simulink model "aero_ground_model"  (R2013b)
settings: Solver=ode23  StartTime=0.0  StopTime=100  FixedStep=0.01  MaxStep=1  RelTol=1e-3
undefined symbols (not defined in the file or in its folder): par
libraries: simulink x12, coeffs x3, lateral_model x3, dspswit3 x1
(part 2 of 2)

== system aero_ground_model/Physical Model/Tire Forces/Wheels Velocity/Velocity_L ==
  STATE : Inport
  " " : Constant  Value=par.l_yL
  "  " : Constant  Value=par.l_xL
  Add : Sum
  Add1 : Sum  Inputs=+-
  Bus Creator : BusCreator  Inputs=2
  Bus Selector : BusSelector  OutputSignals=[Vx; Vy],Wz
  Bus Selector1 : BusSelector  OutputSignals=v_X,v_Y
  Product : Product
  Product1 : Product
  V_L : Outport
  wires:
  STATE/1 -> Bus Selector/1
  Bus Selector/1 -> Bus Selector1/1  "<[Vx; Vy]>"
  Bus Selector1/1 -> Add/1  "<v_X>"
  Bus Selector/2 -> Product1/1, Product/2  "<Wz>"
  " "/1 -> Product/1
  Product/1 -> Add/2
  Product1/1 -> Add1/2
  Bus Selector1/2 -> Add1/1  "<v_Y>"
  "  "/1 -> Product1/2
  Add1/1 -> Bus Creator/2  "V_y"
  Add/1 -> Bus Creator/1  "V_x"
  Bus Creator/1 -> V_L/1

== system aero_ground_model/Physical Model/Tire Forces/Wheels Velocity/Velocity_N ==
  note: V_N = f(V,W)
  note: 1. Vx_N = Vx * cos(delta) + (Vy + l_xN * Wz) * sin(delta)
      |
      | 2. Vy_N = (Vx + l_xN * Wz) * cos(delta) - Vx * sin(delta)
  STATE : Inport
  delta : Inport  Port=2
  Bus Creator : BusCreator  Inputs=2
  Bus Selector : BusSelector  OutputSignals=[Vx; Vy],Wz
  Bus Selector1 : BusSelector  OutputSignals=v_X,v_Y
  VxN : Subsystem
  VyN : Subsystem
  V_N : Outport
  wires:
  STATE/1 -> Bus Selector/1
  Bus Selector/1 -> Bus Selector1/1  "<[Vx; Vy]>"
  VyN/1(VyN) -> Bus Creator/2  "V_y"
  Bus Creator/1 -> V_N/1
  delta/1 -> VyN/1(delta), VxN/1(delta)
  Bus Selector1/1 -> VyN/2(Vx), VxN/2(Vx)  "<v_X>"
  Bus Selector1/2 -> VyN/3(Vy), VxN/3(Vy)  "<v_Y>"
  Bus Selector/2 -> VyN/4(Wz), VxN/4(Wz)  "<Wz>"
  VxN/1(VxN) -> Bus Creator/1  "V_x"

== system aero_ground_model/Physical Model/Tire Forces/Wheels Velocity/Velocity_R ==
  STATE : Inport
  " " : Constant  Value=par.l_yR
  "  " : Constant  Value=par.l_xR
  Add : Sum  Inputs=+-
  Add1 : Sum  Inputs=+-
  Bus Creator : BusCreator  Inputs=2
  Bus Selector : BusSelector  OutputSignals=[Vx; Vy],Wz
  Bus Selector1 : BusSelector  OutputSignals=v_X,v_Y
  Product : Product
  Product1 : Product
  V_R : Outport
  wires:
  STATE/1 -> Bus Selector/1
  Bus Selector/1 -> Bus Selector1/1  "<[Vx; Vy]>"
  Bus Selector1/1 -> Add/1  "<v_X>"
  Bus Selector/2 -> Product1/1, Product/2  "<Wz>"
  " "/1 -> Product/1
  Product/1 -> Add/2
  Product1/1 -> Add1/2
  Bus Selector1/2 -> Add1/1  "<v_Y>"
  "  "/1 -> Product1/2
  Add1/1 -> Bus Creator/2  "V_y"
  Add/1 -> Bus Creator/1  "V_x"
  Bus Creator/1 -> V_R/1

== system aero_ground_model/Physical Model/Forces to Velocities/Velocity/velo_X/F_xN * cos(delta) ==
  F_xN : Inport
  delta : Inport  Port=2
  Projection of nose-wheel resistance force into X axis : Product
  Trigonometric Function : Trigonometry  Operator=cos
  Out1 : Outport
  wires:
  F_xN/1 -> Projection of nose-wheel resistance force into X axis/1
  Trigonometric Function/1 -> Projection of nose-wheel resistance force into X axis/2
  Projection of nose-wheel resistance force into X axis/1 -> Out1/1
  delta/1 -> Trigonometric Function/1

== system aero_ground_model/Physical Model/Forces to Velocities/Velocity/velo_X/F_yN * sin(delta) ==
  delta : Inport
  F_yN : Inport  Port=2
  Projection of nose-wheel lateral force into X-axis : Product
  Trigonometric Function : Trigonometry
  Out1 : Outport
  wires:
  F_yN/1 -> Projection of nose-wheel lateral force into X-axis/1
  Trigonometric Function/1 -> Projection of nose-wheel lateral force into X-axis/2
  Projection of nose-wheel lateral force into X-axis/1 -> Out1/1
  delta/1 -> Trigonometric Function/1

== system aero_ground_model/Physical Model/Forces to Velocities/Velocity/velo_Y/*cos(delta) ==
  delta : Inport
  F_yN : Inport  Port=2
  Projection of nose-wheel lateral force into Y axis : Product
  Trigonometric Function : Trigonometry  Operator=cos
  Out1 : Outport
  wires:
  F_yN/1 -> Projection of nose-wheel lateral force into Y axis/1
  Trigonometric Function/1 -> Projection of nose-wheel lateral force into Y axis/2
  Projection of nose-wheel lateral force into Y axis/1 -> Out1/1
  delta/1 -> Trigonometric Function/1

== system aero_ground_model/Physical Model/Forces to Velocities/Velocity/velo_Y/*sin(delta) ==
  delta : Inport
  F_xN : Inport  Port=2
  Projection of nose-wheel resistance force into Y-axis : Product
  Trigonometric Function : Trigonometry
  Out1 : Outport
  wires:
  Trigonometric Function/1 -> Projection of nose-wheel resistance force into Y-axis/2
  Projection of nose-wheel resistance force into Y-axis/1 -> Out1/1
  delta/1 -> Trigonometric Function/1
  F_xN/1 -> Projection of nose-wheel resistance force into Y-axis/1

== system aero_ground_model/Physical Model/Tire Forces/Lateral tire Force/Slip Angles/arctan(V_L) ==
  note: Slip Angle
  note: alpha = arctan(Vy/Vx)
  V : Inport
  Bus Selector : BusSelector  OutputSignals=V_y,V_x
  Trigonometric Function : Trigonometry  Operator=atan2
  atan(V) : Outport
  wires:
  V/1 -> Bus Selector/1
  Bus Selector/2 -> Trigonometric Function/2  "<V_x>"
  Bus Selector/1 -> Trigonometric Function/1  "<V_y>"
  Trigonometric Function/1 -> atan(V)/1

== system aero_ground_model/Physical Model/Tire Forces/Lateral tire Force/Slip Angles/arctan(V_N) ==
  note: Slip Angle
  note: alpha = arctan(Vy/Vx)
  V : Inport
  Bus Selector : BusSelector  OutputSignals=V_y,V_x
  Trigonometric Function : Trigonometry  Operator=atan2
  atan(V) : Outport
  wires:
  V/1 -> Bus Selector/1
  Bus Selector/2 -> Trigonometric Function/2  "<V_x>"
  Trigonometric Function/1 -> atan(V)/1
  Bus Selector/1 -> Trigonometric Function/1  "<V_y>"

== system aero_ground_model/Physical Model/Tire Forces/Lateral tire Force/Slip Angles/arctan(V_R) ==
  note: Slip Angle
  note: alpha = arctan(Vy/Vx)
  V : Inport
  Bus Selector : BusSelector  OutputSignals=V_y,V_x
  Trigonometric Function : Trigonometry  Operator=atan2
  atan(V) : Outport
  wires:
  V/1 -> Bus Selector/1
  Bus Selector/2 -> Trigonometric Function/2  "<V_x>"
  Trigonometric Function/1 -> atan(V)/1
  Bus Selector/1 -> Trigonometric Function/1  "<V_y>"

== system aero_ground_model/Physical Model/Tire Forces/Longitudal Tire Force/Braking/L brake ==
  note: brakes - ratio of brakes being applied (0-1)
      | mu_Beff - friction coeff., effectivity of ABS braking system
  note: Model of simple ABS brakes
  F_zRL : Inport
  environ : Inport  Port=2
  brakes : Inport  Port=3
  Bus Selector : BusSelector  OutputSignals=coeffs_L.mu_Beff
  Gain : Gain  Gain=0.3
  Product : Product
  Product1 : Product
  F_xL : Outport
  wires:
  environ/1 -> Bus Selector/1
  Bus Selector/1 -> Product/2  "<mu_Beff>"
  F_zRL/1 -> Product/1
  brakes/1 -> Product1/1
  Product/1 -> Product1/2
  Product1/1 -> Gain/1
  Gain/1 -> F_xL/1

== system aero_ground_model/Physical Model/Tire Forces/Longitudal Tire Force/Braking/R brake ==
  note: brakes - ratio of brakes being applied (0-1)
      | mu_Beff - friction coeff., effectivity of ABS braking system
  note: Model of simple ABS brakes
  brakes : Inport
  F_zRL : Inport  Port=2
  environ : Inport  Port=3
  Bus Selector : BusSelector  OutputSignals=coeffs_R.mu_Beff
  Gain : Gain  Gain=0.3
  Product : Product
  Product1 : Product
  F_xR : Outport
  wires:
  environ/1 -> Bus Selector/1
  Bus Selector/1 -> Product/2  "<mu_Beff>"
  F_zRL/1 -> Product/1
  Product/1 -> Product1/2
  brakes/1 -> Product1/1
  Product1/1 -> Gain/1
  Gain/1 -> F_xR/1

== system aero_ground_model/Physical Model/Tire Forces/Longitudal Tire Force/Rolling Resistance/Resist_L ==
  note: F_xL = mu_R * F_zL * (vL / v_thresh)
  note: Rolling Resistance of Left Tire
  coeffs : Inport
  F_zL : Inport  Port=2
  Bus Selector : BusSelector  OutputSignals=mu_R
  Product : Product
  F_xL : Outport
  wires:
  F_zL/1 -> Product/1
  Bus Selector/1 -> Product/2  "<mu_R>"
  coeffs/1 -> Bus Selector/1
  Product/1 -> F_xL/1

== system aero_ground_model/Physical Model/Tire Forces/Longitudal Tire Force/Rolling Resistance/Resist_N ==
  note: F_xN = mu_R * F_zN * (v / v_thresh)
  note: Rolling Resistance of Nose-Wheel Tire
  F_zN : Inport
  coeffs : Inport  Port=2
  Bus Selector : BusSelector  OutputSignals=mu_R
  Product : Product
  F_xN : Outport
  wires:
  F_zN/1 -> Product/1
  Bus Selector/1 -> Product/2  "<mu_R>"
  coeffs/1 -> Bus Selector/1
  Product/1 -> F_xN/1

== system aero_ground_model/Physical Model/Tire Forces/Longitudal Tire Force/Rolling Resistance/Resist_R ==
  note: (vR / v_thresh) limited to range 0-1
      | used to eliminate resistance forces
      | when plane stands still
  note: F_xR = mu_R * F_zR * (vR / v_thresh)
  note: Rolling Resistance of Right Tire
  F_zR : Inport
  coeffs : Inport  Port=2
  Bus Selector : BusSelector  OutputSignals=mu_R
  Product : Product
  F_xR : Outport
  wires:
  F_zR/1 -> Product/1
  Bus Selector/1 -> Product/2  "<mu_R>"
  coeffs/1 -> Bus Selector/1
  Product/1 -> F_xR/1

== system aero_ground_model/Physical Model/Tire Forces/Wheels Velocity/Velocity_N/VxN ==
  delta : Inport
  Vx : Inport  Port=2
  Vy : Inport  Port=3
  Wz : Inport  Port=4
  "     " : Constant  Value=par.l_xN
  Add : Sum
  Add2 : Sum
  Gain1 : Gain  Commented=on  Gain=-1
  Product1 : Product
  Product2 : Product
  Product3 : Product
  Trigonometric Function : Trigonometry  Operator=cos
  Trigonometric Function1 : Trigonometry
  VxN : Outport
  wires:
  Product3/1 -> Add/2
  Add/1 -> VxN/1  "V_x"
  Add2/1 -> Product3/2
  delta/1 -> Trigonometric Function/1, Trigonometric Function1/1
  Wz/1 -> Product1/2
  Product2/1 -> Add/1
  Trigonometric Function1/1 -> Product3/1
  Product1/1 -> Add2/2
  "     "/1 -> Product1/1
  Trigonometric Function/1 -> Product2/2
  Vx/1 -> Product2/1
  Vy/1 -> Add2/1

== system aero_ground_model/Physical Model/Tire Forces/Wheels Velocity/Velocity_N/VyN ==
  delta : Inport
  Vx : Inport  Port=2
  Vy : Inport  Port=3
  Wz : Inport  Port=4
  "     " : Constant  Value=par.l_xN
  Add : Sum  Inputs=-+
  Add2 : Sum
  Product1 : Product
  Product2 : Product
  Product3 : Product
  Trigonometric Function : Trigonometry
  Trigonometric Function1 : Trigonometry  Operator=cos
  VyN : Outport
  wires:
  Vy/1 -> Add2/1
  Product3/1 -> Add/2
  Add/1 -> VyN/1  "V_y"
  Add2/1 -> Product3/2
  delta/1 -> Trigonometric Function/1, Trigonometric Function1/1
  Wz/1 -> Product1/2
  Product2/1 -> Add/1
  Trigonometric Function1/1 -> Product3/1
  Product1/1 -> Add2/2
  "     "/1 -> Product1/1
  Trigonometric Function/1 -> Product2/2
  Vx/1 -> Product2/1

== matlab function aero_ground_model/Direction control/Target selector/Targets/target selector X ==
  data: vals input; target output; idx input
function target  = select(vals, idx)
%#codegen

%selects specified element from array of targets
%http://www.mathworks.com/help/simulink/ug/creating-an-example-model-that-uses-a-matlab-function-block.html
%if idx out of range select first/last
if idx < 1
    idx = 1;
end    

len = length(vals);
if idx <= len
   target = vals(idx); 
else
   target = vals(len);
end

== matlab function aero_ground_model/Direction control/Target selector/Targets/target selector Y ==
  data: vals input; target output; idx input
function target  = select(vals, idx)
%#codegen

%selects specified element from array of targets
%if idx out of range select first/last

if idx < 1
    idx = 1;
end 

len = length(vals);
if idx <= len
   target = vals(idx); 
else
   target = vals(len);
end
